simulink model "battery_model_2RC"  (R2015a)
settings: Solver=ode1  StartTime=min(Mess.time)  StopTime=max(Mess.time)  FixedStep=Mess.time(2)-Mess.time(1)  MaxStep=0.1  RelTol=1e-8
values from neighbouring files (symbols this model uses):
  Cn = str2double(Cn{1})    [main.m]
  OCV =     [OCV.mat]    (also in main.m = simResultsVoltage.signals.values(:,3))
  SOC = [30, 60, 80]    [Compariosn_between_resistances_charge_and_discharge.m]    (also in Experiment_1_Task_4_batteryC_OCV_curve.m = linspace(0, 100, 11); Task_3_2__C_ResistanceVSSOC.m; Task_3_2__Discharge_ResistanceVSSOC.m; Task_3_3_EfficiencyVSSOC.m)
  SOC_0 = str2double(SOC_0{1})    [main.m]
  Strom = [-2 -1]    [main.m]
  Stromprofil = str2double(Stromprofil{1})    [main.m]
undefined symbols (not defined in the file or in its folder): Cion1, Cion2, Rion1, Rion2, Rohm
CloseFcn:
  | rtwprivate ssgencode ModelCloseRequest erstesmodell
settings Model: NumberOfSteps=1000  Creator=SYSEAEB  LastModifiedBy=hofmann
settings SolverCC: InitialStep=0.00001  MaxConsecutiveMinStep=1000  ZeroCrossAlgorithm=Adaptive  AutoInsertRateTranBlk=on
settings DataIOCC: LimitDataPoints=off  SignalLoggingSaveFormat=ModelDataLogs
settings OptimizationCC: ExpressionDepthLimit=2147483647
settings DebuggingCC: AlgebraicLoopMsg=none  UnderspecifiedInitializationDetection=Classic  MergeDetectMultiDrivingBlocksExec=none  FcnCallInpInsideContextMsg=EnableAllAsWarning  UniqueDataStoreMsg=warning  StateNameClashWarn=warning
settings SFSimCC: SimParseCustomCode=off
settings GRTTargetCC: CombineOutputUpdateFcns=off  GRTInterface=on

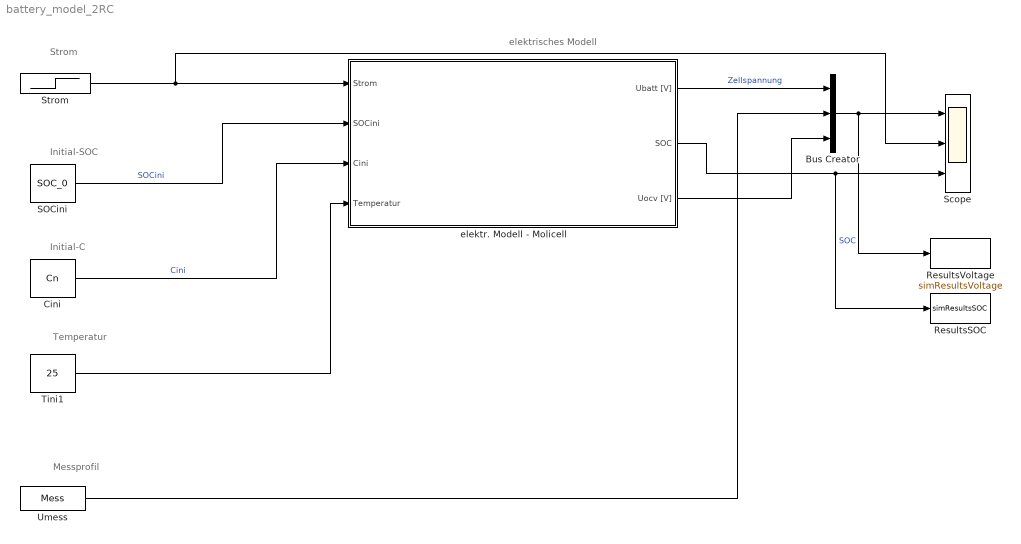
== system battery_model_2RC ==
  note: Strom
  note: Initial-SOC
  note: Initial-C
  note: elektrisches Modell
  note: Temperatur
  note: Messprofil
  Bus Creator : BusCreator  Inputs=3
  Cini : Constant  Value=Cn  SampleTime=-1
  ResultsSOC : ToWorkspace  VariableName=simResultsSOC  SaveFormat=Structure With Time  SampleTime=-1
  ResultsVoltage : ToWorkspace  VariableName=simResultsVoltage  SaveFormat=Structure With Time  SampleTime=-1
  SOCini : Constant  Value=SOC_0  SampleTime=-1
  Scope : Scope  NumInputPorts=3
      settings: TimeRange=0.002000039999999981  MaxDataPoints=5000  SaveToWorkspace=off  SaveName=ScopeData3  YMin=3.3~3.3~3.3  YMax=3.7~3.7~3.7  SampleTime=-1  DataFormat=Array
  Strom : Step  Time=0  After=Stromprofil
  Tini1 : Constant  Value=25  SampleTime=-1
  Umess : FromWorkspace  VariableName=Mess  OutputAfterFinalValue=Holding final value
  elektr. Modell - Molicell : Subsystem
  wires:
  Tini1/1 -> elektr. Modell - Molicell/4(Temperatur)
  SOCini/1 -> elektr. Modell - Molicell/2(SOCini)  "SOCini"
  Cini/1 -> elektr. Modell - Molicell/3(Cini)  "Cini"
  Bus Creator/1 -> ResultsVoltage/1, Scope/1
  elektr. Modell - Molicell/1(Ubatt [V]) -> Bus Creator/1  "Zellspannung"
  elektr. Modell - Molicell/3(Uocv [V]) -> Bus Creator/3
  elektr. Modell - Molicell/2(SOC) -> ResultsSOC/1, Scope/3  "SOC"
  Strom/1 -> Scope/2, elektr. Modell - Molicell/1(Strom)
  Umess/1 -> Bus Creator/2

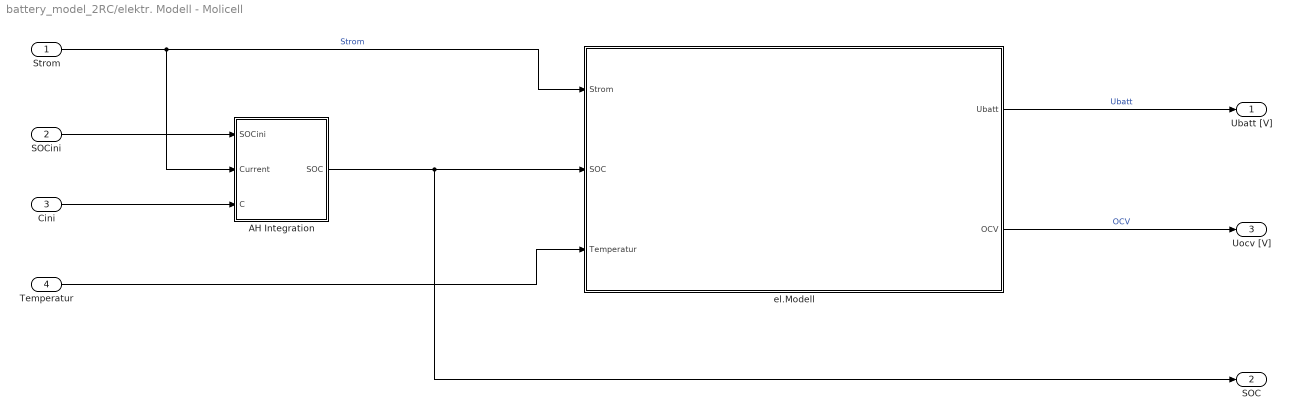
== system battery_model_2RC/elektr. Modell - Molicell ==
  Strom : Inport
  SOCini : Inport  Port=2
  Cini : Inport  Port=3
  Temperatur : Inport  Port=4
  AH Integration : Subsystem
  el.Modell : Subsystem  TreatAsAtomicUnit=on
  Ubatt [V] : Outport
  SOC : Outport  Port=2
  Uocv [V] : Outport  Port=3
  wires:
  SOCini/1 -> AH Integration/1(SOCini)
  Cini/1 -> AH Integration/3(C)
  AH Integration/1(SOC) -> SOC/1, el.Modell/2(SOC)
  Temperatur/1 -> el.Modell/3(Temperatur)
  el.Modell/1(Ubatt) -> Ubatt [V]/1  "Ubatt"
  el.Modell/2(OCV) -> Uocv [V]/1  "OCV"
  Strom/1 -> AH Integration/2(Current), el.Modell/1(Strom)  "Strom"

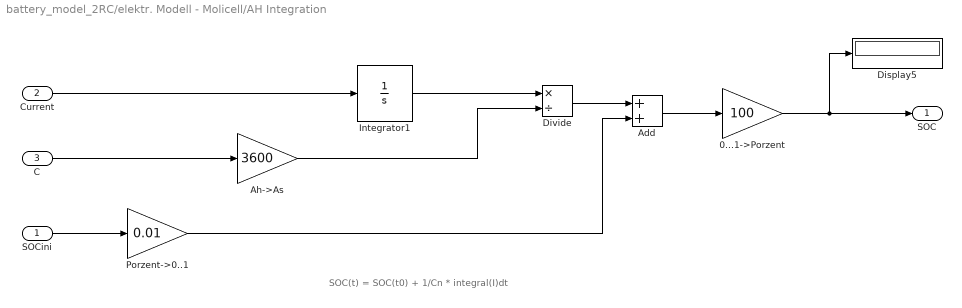
== system battery_model_2RC/elektr. Modell - Molicell/AH Integration ==
  note: SOC(t) = SOC(t0) + 1/Cn * integral(I)dt
  SOCini : Inport
  Current : Inport  Port=2
  C : Inport  Port=3
  0...1->Porzent : Gain  Gain=100
  Add : Sum
  Ah->As : Gain  Gain=3600
  Display5 : Display
  Divide : Product  Inputs=*/
  Integrator1 : Integrator  ZeroCross=off
  Porzent->0..1 : Gain  Gain=0.01
  SOC : Outport
  wires:
  SOCini/1 -> Porzent->0..1/1
  C/1 -> Ah->As/1
  Integrator1/1 -> Divide/1
  Ah->As/1 -> Divide/2
  Divide/1 -> Add/1
  Porzent->0..1/1 -> Add/2
  Add/1 -> 0...1->Porzent/1
  0...1->Porzent/1 -> SOC/1, Display5/1
  Current/1 -> Integrator1/1

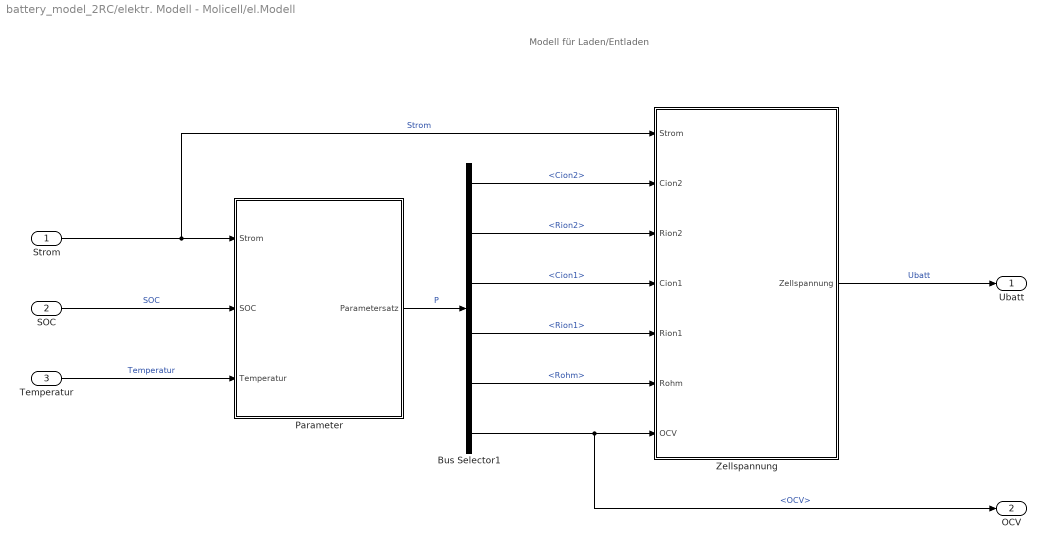
== system battery_model_2RC/elektr. Modell - Molicell/el.Modell ==
  note: Modell für Laden/Entladen
  Strom : Inport
  SOC : Inport  Port=2
  Temperatur : Inport  Port=3
  Bus Selector1 : BusSelector  OutputSignals=Cion2,Rion2,Cion1,Rion1,Rohm,OCV
  Parameter : Subsystem
  Zellspannung : Subsystem
  Ubatt : Outport
  OCV : Outport  Port=2
  wires:
  Zellspannung/1(Zellspannung) -> Ubatt/1  "Ubatt"
  Strom/1 -> Zellspannung/1(Strom), Parameter/1(Strom)  "Strom"
  SOC/1 -> Parameter/2(SOC)  "SOC"
  Temperatur/1 -> Parameter/3(Temperatur)  "Temperatur"
  Bus Selector1/1 -> Zellspannung/2(Cion2)  "<Cion2>"
  Bus Selector1/2 -> Zellspannung/3(Rion2)  "<Rion2>"
  Bus Selector1/3 -> Zellspannung/4(Cion1)  "<Cion1>"
  Bus Selector1/4 -> Zellspannung/5(Rion1)  "<Rion1>"
  Bus Selector1/5 -> Zellspannung/6(Rohm)  "<Rohm>"
  Bus Selector1/6 -> OCV/1, Zellspannung/7(OCV)  "<OCV>"
  Parameter/1(Parametersatz) -> Bus Selector1/1  "P"

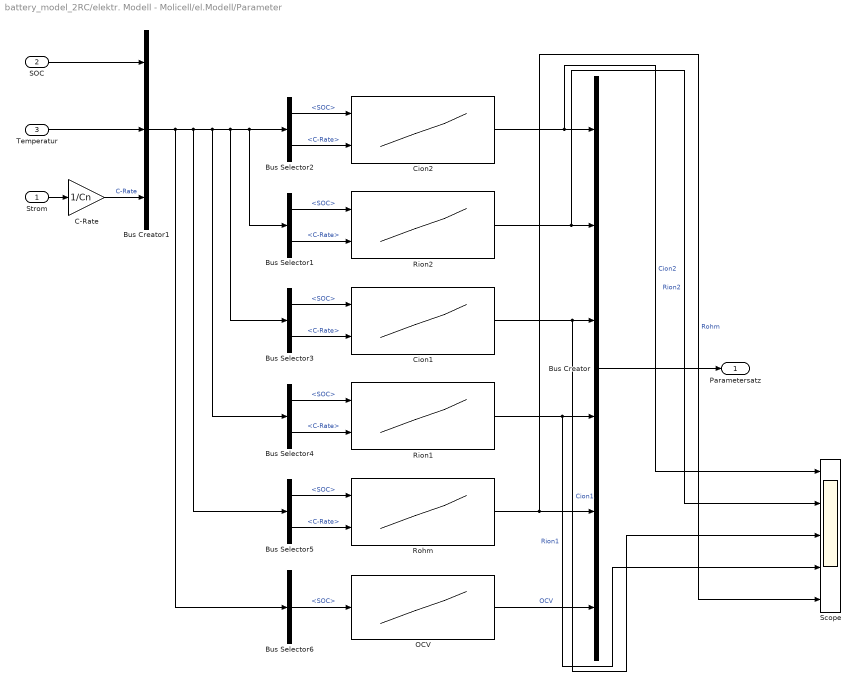
== system battery_model_2RC/elektr. Modell - Molicell/el.Modell/Parameter ==
  Strom : Inport
  SOC : Inport  Port=2
  Temperatur : Inport  Port=3
  Bus Creator : BusCreator  Inputs=6
  Bus Creator1 : BusCreator  Inputs=3
  Bus Selector{1..5} (5 alike) : BusSelector  OutputSignals=SOC,C-Rate
  Bus Selector6 : BusSelector  OutputSignals=SOC
  C-Rate : Gain  Gain=1/Cn
  Cion1 : Lookup_n-D  BreakpointsForDimension1=SOC  BreakpointsForDimension2=Strom  BreakpointsForDimension3=Strom  Table=Cion1  ExtrapMethod=Clip  RndMeth=Simplest  InputSameDT=on
  Cion2 : Lookup_n-D  BreakpointsForDimension1=SOC  BreakpointsForDimension2=Strom  BreakpointsForDimension3=Strom  Table=Cion2  ExtrapMethod=Clip  RndMeth=Simplest  InputSameDT=on
  OCV : Lookup_n-D  NumberOfTableDimensions=1  BreakpointsForDimension1=OCV(:,1)  BreakpointsForDimension2=[1:3]  Table=OCV(:,2)  ExtrapMethod=Clip  RndMeth=Simplest  InputSameDT=on
  Rion1 : Lookup_n-D  BreakpointsForDimension1=SOC  BreakpointsForDimension2=Strom  BreakpointsForDimension3=Strom  Table=Rion1  ExtrapMethod=Clip  RndMeth=Simplest  InputSameDT=on
  Rion2 : Lookup_n-D  BreakpointsForDimension1=SOC  BreakpointsForDimension2=Strom  BreakpointsForDimension3=Strom  Table=Rion2  ExtrapMethod=Clip  RndMeth=Simplest  InputSameDT=on
  Rohm : Lookup_n-D  BreakpointsForDimension1=SOC  BreakpointsForDimension2=Strom  BreakpointsForDimension3=Strom  Table=Rohm  ExtrapMethod=Clip  RndMeth=Simplest  InputSameDT=on
  Scope : Scope  NumInputPorts=5
      settings: TimeRange=auto  LimitDataPoints=on  MaxDataPoints=5000  SaveToWorkspace=off  SaveName=ScopeData2  YMin=239.917~239.917~239.917~239.917~239.917  YMax=239.922~239.922~239.922~239.922~239.922  SampleTime=-1  DataFormat=Array
  Parametersatz : Outport
  wires:
  SOC/1 -> Bus Creator1/1
  Temperatur/1 -> Bus Creator1/2
  Bus Selector2/1 -> Cion2/1  "<SOC>"
  Bus Selector6/1 -> OCV/1  "<SOC>"
  OCV/1 -> Bus Creator/6  "OCV"
  Cion2/1 -> Scope/1, Bus Creator/1  "Cion2"
  Rion2/1 -> Scope/2, Bus Creator/2  "Rion2"
  Cion1/1 -> Scope/3, Bus Creator/3  "Cion1"
  Rion1/1 -> Scope/4, Bus Creator/4  "Rion1"
  Rohm/1 -> Scope/5, Bus Creator/5  "Rohm"
  Bus Selector2/2 -> Cion2/2  "<C-Rate>"
  Bus Selector1/1 -> Rion2/1  "<SOC>"
  Bus Selector1/2 -> Rion2/2  "<C-Rate>"
  Bus Selector3/1 -> Cion1/1  "<SOC>"
  Bus Selector3/2 -> Cion1/2  "<C-Rate>"
  Bus Selector4/1 -> Rion1/1  "<SOC>"
  Bus Selector4/2 -> Rion1/2  "<C-Rate>"
  Bus Selector5/1 -> Rohm/1  "<SOC>"
  Bus Selector5/2 -> Rohm/2  "<C-Rate>"
  Bus Creator1/1 -> Bus Selector6/1, Bus Selector5/1, Bus Selector4/1, Bus Selector3/1, Bus Selector2/1, Bus Selector1/1
  Bus Creator/1 -> Parametersatz/1
  Strom/1 -> C-Rate/1
  C-Rate/1 -> Bus Creator1/3  "C-Rate"

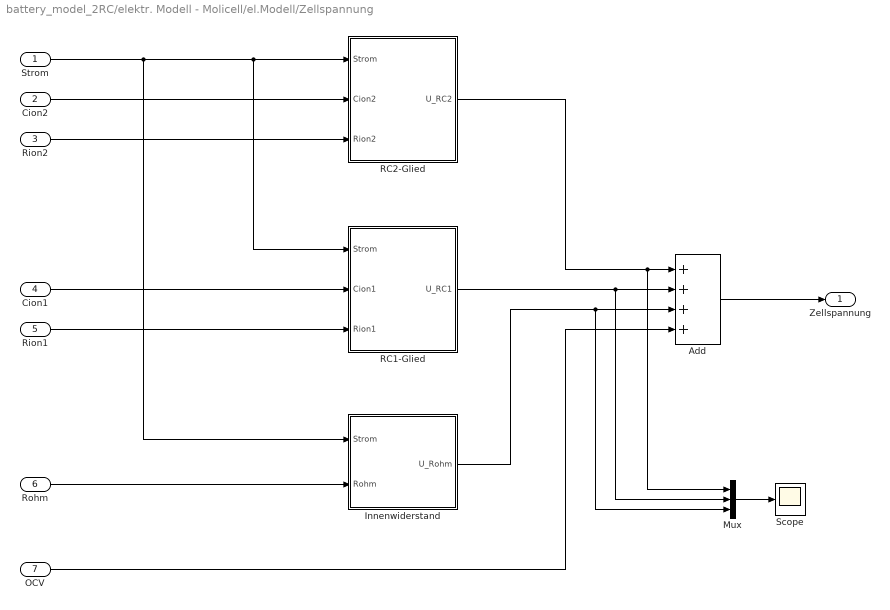
== system battery_model_2RC/elektr. Modell - Molicell/el.Modell/Zellspannung ==
  Strom : Inport
  Cion2 : Inport  Port=2
  Rion2 : Inport  Port=3
  Cion1 : Inport  Port=4
  Rion1 : Inport  Port=5
  Rohm : Inport  Port=6
  OCV : Inport  Port=7
  Add : Sum  Inputs=++++
  Innenwiderstand : Subsystem
  Mux : Mux  Inputs=3
  RC1-Glied : Subsystem
  RC2-Glied : Subsystem
  Scope : Scope
      settings: TimeRange=auto  LimitDataPoints=on  MaxDataPoints=5000  SaveToWorkspace=off  YMin=-10  YMax=10  SampleTime=-1  DataFormat=Array
  Zellspannung : Outport
  wires:
  Rion2/1 -> RC2-Glied/3(Rion2)
  Cion2/1 -> RC2-Glied/2(Cion2)
  Rohm/1 -> Innenwiderstand/2(Rohm)
  OCV/1 -> Add/4
  Rion1/1 -> RC1-Glied/3(Rion1)
  Cion1/1 -> RC1-Glied/2(Cion1)
  Innenwiderstand/1(U_Rohm) -> Mux/3, Add/3
  RC1-Glied/1(U_RC1) -> Mux/2, Add/2
  RC2-Glied/1(U_RC2) -> Mux/1, Add/1
  Add/1 -> Zellspannung/1
  Strom/1 -> RC1-Glied/1(Strom), RC2-Glied/1(Strom), Innenwiderstand/1(Strom)
  Mux/1 -> Scope/1

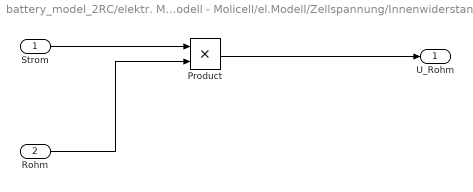
== system battery_model_2RC/elektr. Modell - Molicell/el.Modell/Zellspannung/Innenwiderstand ==
  Strom : Inport
  Rohm : Inport  Port=2
  Product : Product  RndMeth=Zero
  U_Rohm : Outport
  wires:
  Strom/1 -> Product/1
  Rohm/1 -> Product/2
  Product/1 -> U_Rohm/1

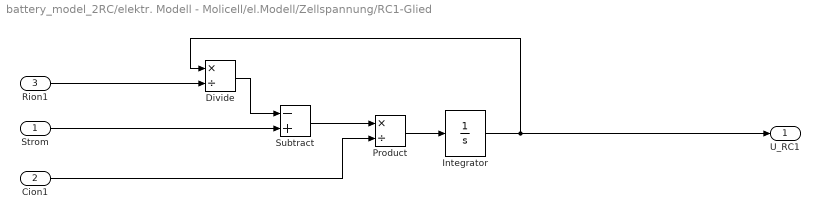
== system battery_model_2RC/elektr. Modell - Molicell/el.Modell/Zellspannung/RC1-Glied ==
  Strom : Inport
  Cion1 : Inport  Port=2
  Rion1 : Inport  Port=3
  Divide : Product  Inputs=*/
  Integrator : Integrator  UpperSaturationLimit=1  LowerSaturationLimit=-1  ZeroCross=off
  Product : Product  Inputs=*/  RndMeth=Zero
  Subtract : Sum  Inputs=-+
  U_RC1 : Outport
  wires:
  Integrator/1 -> Divide/1, U_RC1/1
  Divide/1 -> Subtract/1
  Strom/1 -> Subtract/2
  Subtract/1 -> Product/1
  Product/1 -> Integrator/1
  Cion1/1 -> Product/2
  Rion1/1 -> Divide/2

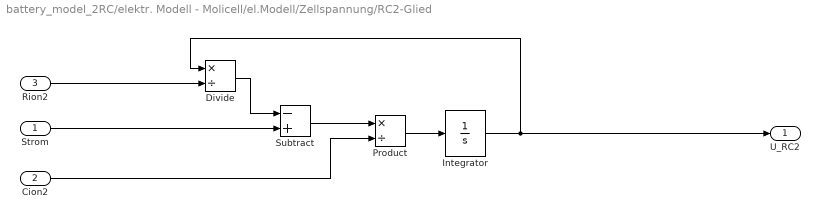
== system battery_model_2RC/elektr. Modell - Molicell/el.Modell/Zellspannung/RC2-Glied ==
  Strom : Inport
  Cion2 : Inport  Port=2
  Rion2 : Inport  Port=3
  Divide : Product  Inputs=*/
  Integrator : Integrator  ZeroCross=off
  Product : Product  Inputs=*/  RndMeth=Zero
  Subtract : Sum  Inputs=-+
  U_RC2 : Outport
  wires:
  Integrator/1 -> Divide/1, U_RC2/1
  Divide/1 -> Subtract/1
  Strom/1 -> Subtract/2
  Subtract/1 -> Product/1
  Cion2/1 -> Product/2
  Product/1 -> Integrator/1
  Rion2/1 -> Divide/2
